simulink model "simscap_Mech1"  (R2015a)
settings: Solver=ode45  StartTime=0.0  StopTime=3  RelTol=1e-3
undefined symbols (not defined in the file or in its folder): Bj, Bp, Mj, Mp
libraries: fl_lib x15, nesl_utility x7
settings Model: Creator=ahmed alaa  LastModifiedBy=ahmed alaa

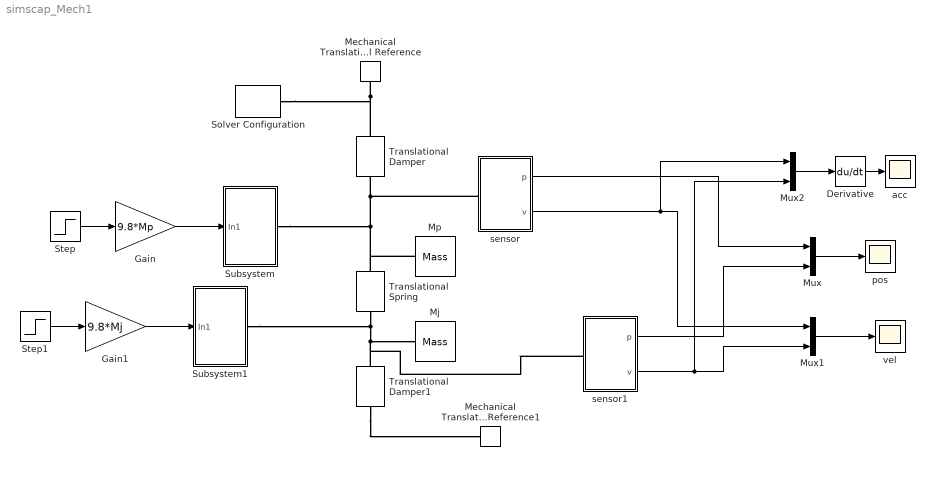
== system simscap_Mech1 ==
  Derivative : Derivative
  Gain : Gain  Gain=9.8*Mp
  Gain1 : Gain  Gain=9.8*Mj
  Mechanical Translational Reference : fl_lib/Mechanical/Translational Elements/Mechanical Translational Reference
  Mechanical Translational Reference1 : fl_lib/Mechanical/Translational Elements/Mechanical Translational Reference
  Mj : fl_lib/Mechanical/Translational Elements/Mass  mass=Mj kg  v_specify=on  v_priority=High  v=20 m/s  f_specify=off  f_priority=High  f=0 N
  Mp : fl_lib/Mechanical/Translational Elements/Mass  mass=Mp kg  v_specify=on  v_priority=High  v=20 m/s  f_specify=off  f_priority=High  f=0 N
  Mux : Mux  Inputs=2
  Mux1 : Mux  Inputs=2
  Mux2 : Mux  Inputs=2
  Solver Configuration : nesl_utility/Solver Configuration  PhysicalDomain=network_engine_domain  SubClassName=solver  LeftPortType=input  RightPortType=generic  Accelerate=off  Tones=[]  Harmonics=[]  SimulateNoise=off  Profile=off  UseLocalSampling=off  EnableSwitchedLinearOptims=on  FrequencyDomain=off  UseCCode=off  RelTol=0.001  AbsTol=1e-06  MinStep=1e-09  ToWorkspace=off  RevertToSquareIcSolve=off  NumHomotopyIterations=100  DoDC=off  ResidualTolerance=1e-09  UseLocalSolver=off  LocalSolverChoice=NE_BACKWARD_EULER_ADVANCER  LocalSolverSampleTime=0.001  DoFixedCost=off  MaxNonlinIter=3  MaxModeIter=2  LinearAlgebra=Sparse  DelaysMemoryBudget=1024  AutomaticFiltering=on  FilteringTimeConstant=0.001
  Step : Step  Time=0  SampleTime=0
  Step1 : Step  Time=0  SampleTime=0
  Subsystem : Subsystem
  Subsystem1 : Subsystem
  Translational Damper : fl_lib/Mechanical/Translational Elements/Translational Damper  D=Bp N/(m/s)  v_specify=off  v_priority=High  v=0 m/s  f_specify=off  f_priority=High  f=0 N
  Translational Damper1 : fl_lib/Mechanical/Translational Elements/Translational Damper  D=Bj N/(m/s)  v_specify=off  v_priority=High  v=0 m/s  f_specify=off  f_priority=High  f=0 N
  Translational Spring : fl_lib/Mechanical/Translational Elements/Translational Spring  spr_rate=Kr N/m  v_specify=off  v_priority=High  v=0 m/s  f_specify=off  f_priority=High  f=0 N  x_specify=off  x_priority=High  x=0 m
  acc : Scope
      settings: SaveName=ScopeData2
  pos : Scope
  sensor : Subsystem
  sensor1 : Subsystem
  vel : Scope
  wires:
  Step/1 -> Gain/1
  Gain/1 -> Subsystem/1(In1)
  Step1/1 -> Gain1/1
  Gain1/1 -> Subsystem1/1(In1)
  sensor/1(p) -> Mux/1
  sensor1/1(p) -> Mux/2
  Mux/1 -> pos/1
  Mux1/1 -> vel/1
  sensor/2(v) -> Mux2/1, Mux1/1
  sensor1/2(v) -> Mux2/2, Mux1/2
  Mux2/1 -> Derivative/1
  Derivative/1 -> acc/1
  connections:
  Mechanical Translational Reference/LConn1 -- Translational Damper/LConn1 -- Solver Configuration/RConn1
  sensor/LConn1 -- Subsystem/RConn1 -- Translational Spring/LConn1 -- Mp/LConn1 -- Translational Damper/RConn1
  Translational Spring/RConn1 -- Subsystem1/RConn1 -- sensor1/LConn1 -- Translational Damper1/LConn1 -- Mj/LConn1
  Translational Damper1/RConn1 -- Mechanical Translational Reference1/LConn1

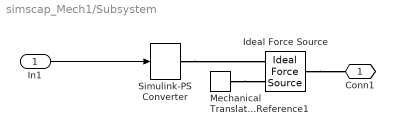
== system simscap_Mech1/Subsystem ==
  In1 : Inport
  Ideal Force Source : fl_lib/Mechanical/Mechanical Sources/Ideal Force Source
  Mechanical Translational Reference1 : fl_lib/Mechanical/Translational Elements/Mechanical Translational Reference
  Simulink-PS Converter : nesl_utility/Simulink-PS Converter  PhysicalDomain=network_engine_domain  SubClassName=ps_input  LeftPortType=input  RightPortType=output  PseudoPeriodic=off  Frequencies=[]  NoiseDistribution=none  NoiseParameters=[]  Unit=1  AffineConversion=off  InputFiltering=off  SimscapeFilterOrder=1  InputFilterTimeConstant=0.001  UdotUserProvided=1
  Conn1 : PMIOPort  Port=1  Side=Right
  wires:
  In1/1 -> Simulink-PS Converter/1
  connections:
  Mechanical Translational Reference1/LConn1 -- Ideal Force Source/RConn2
  Simulink-PS Converter/RConn1 -- Ideal Force Source/RConn1
  Ideal Force Source/LConn1 -- Conn1/RConn1

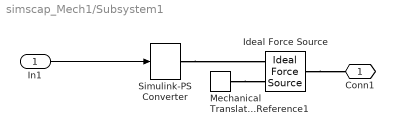
== system simscap_Mech1/Subsystem1 ==
  In1 : Inport
  Ideal Force Source : fl_lib/Mechanical/Mechanical Sources/Ideal Force Source
  Mechanical Translational Reference1 : fl_lib/Mechanical/Translational Elements/Mechanical Translational Reference
  Simulink-PS Converter : nesl_utility/Simulink-PS Converter  PhysicalDomain=network_engine_domain  SubClassName=ps_input  LeftPortType=input  RightPortType=output  PseudoPeriodic=off  Frequencies=[]  NoiseDistribution=none  NoiseParameters=[]  Unit=1  AffineConversion=off  InputFiltering=off  SimscapeFilterOrder=1  InputFilterTimeConstant=0.001  UdotUserProvided=1
  Conn1 : PMIOPort  Port=1  Side=Right
  wires:
  In1/1 -> Simulink-PS Converter/1
  connections:
  Ideal Force Source/LConn1 -- Conn1/RConn1
  Simulink-PS Converter/RConn1 -- Ideal Force Source/RConn1
  Mechanical Translational Reference1/LConn1 -- Ideal Force Source/RConn2

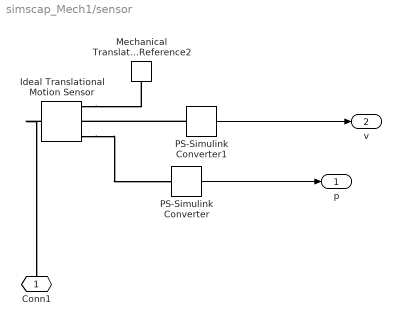
== system simscap_Mech1/sensor ==
  Ideal Translational Motion Sensor : fl_lib/Mechanical/Mechanical Sensors/Ideal Translational Motion Sensor  offset=0 m
  Mechanical Translational Reference2 : fl_lib/Mechanical/Translational Elements/Mechanical Translational Reference
  PS-Simulink Converter : nesl_utility/PS-Simulink Converter  PhysicalDomain=network_engine_domain  SubClassName=ps_output  LeftPortType=input  RightPortType=output  PseudoPeriodic=off  Frequencies=[]  Unit=1  AffineConversion=off
  PS-Simulink Converter1 : nesl_utility/PS-Simulink Converter  PhysicalDomain=network_engine_domain  SubClassName=ps_output  LeftPortType=input  RightPortType=output  PseudoPeriodic=off  Frequencies=[]  Unit=1  AffineConversion=off
  Conn1 : PMIOPort  Port=1  Side=Left
  p : Outport
  v : Outport  Port=2
  wires:
  PS-Simulink Converter/1 -> p/1
  PS-Simulink Converter1/1 -> v/1
  connections:
  PS-Simulink Converter1/LConn1 -- Ideal Translational Motion Sensor/RConn2
  Ideal Translational Motion Sensor/RConn3 -- PS-Simulink Converter/LConn1
  Ideal Translational Motion Sensor/RConn1 -- Mechanical Translational Reference2/LConn1
  Ideal Translational Motion Sensor/LConn1 -- Conn1/RConn1

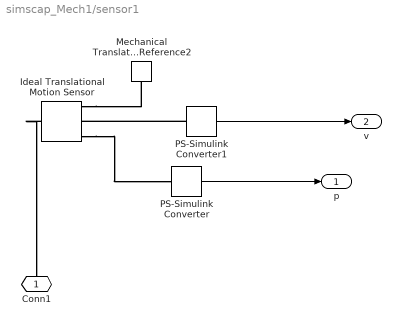
== system simscap_Mech1/sensor1 ==
  Ideal Translational Motion Sensor : fl_lib/Mechanical/Mechanical Sensors/Ideal Translational Motion Sensor  offset=0 m
  Mechanical Translational Reference2 : fl_lib/Mechanical/Translational Elements/Mechanical Translational Reference
  PS-Simulink Converter : nesl_utility/PS-Simulink Converter  PhysicalDomain=network_engine_domain  SubClassName=ps_output  LeftPortType=input  RightPortType=output  PseudoPeriodic=off  Frequencies=[]  Unit=1  AffineConversion=off
  PS-Simulink Converter1 : nesl_utility/PS-Simulink Converter  PhysicalDomain=network_engine_domain  SubClassName=ps_output  LeftPortType=input  RightPortType=output  PseudoPeriodic=off  Frequencies=[]  Unit=1  AffineConversion=off
  Conn1 : PMIOPort  Port=1  Side=Left
  p : Outport
  v : Outport  Port=2
  wires:
  PS-Simulink Converter1/1 -> v/1
  PS-Simulink Converter/1 -> p/1
  connections:
  Ideal Translational Motion Sensor/LConn1 -- Conn1/RConn1
  Ideal Translational Motion Sensor/RConn1 -- Mechanical Translational Reference2/LConn1
  Ideal Translational Motion Sensor/RConn3 -- PS-Simulink Converter/LConn1
  PS-Simulink Converter1/LConn1 -- Ideal Translational Motion Sensor/RConn2
